simulink model "ev"  (R2021a)
settings: Solver=ode4  StartTime=0  StopTime=1082  FixedStep=sim_dt  RelTol=1e-3
model workspace (MAT data in the model file):
  T_eff_bp = [-270; -210; -150; -90; -30; 30; 90; 150; 210; 270]
  T_eff_bp_2 = [-270; -210; -150; -90; -30; 30; 90; 150; 210; 270]
  losses_table = [108927.107777 7820.2782368 7820.17609997 7820.2782368 7820.2782368 7820.2782368 7820.2782368 7820.26172359 7820.2782368 9345.38006027 108927.107777 7820.2782368 ... (100 elements, 10x10)]
  losses_table_2 = [108927.107777 7820.2782368 7820.17609997 7820.2782368 7820.2782368 7820.2782368 7820.2782368 7820.26172359 7820.2782368 9345.38006027 108927.107777 7820.2782368 ... (100 elements, 10x10)]
  w_eff_bp = [0; 888.888888889; 1777.77777778; 2666.66666667; 3555.55555556; 4444.44444444; 5333.33333333; 6222.22222222; 7111.11111111; 8000]
  w_eff_bp_2 = [0; 888.888888889; 1777.77777778; 2666.66666667; 3555.55555556; 4444.44444444; 5333.33333333; 6222.22222222; 7111.11111111; 8000]
undefined symbols (not defined in the file): Af, alpha, Bt, C, C_fa, C_free, C_sa_bat, C_sa_uc, Cd, Cmax, Continuous, Crr, DoD, effi, etaFD, etaG, FD, G, gear, Iucmax, m, M1m, M2m, Max, npar, npar_free, npara, nparf, nparfa, nparsa_bat, nparsa_UC, nser, nser_free, nserfa, nsersa_bat, nsersa_UC, Qbat, regenmax, Ri_BP, RL, ro, Rsc, Rsc_A, Rsc_F, Rsc_sa_bat, Rsc_sa_uc, rw, sim_dt, SOC_BP, SoCbatmax, SoCbatmin, SoCucmax, SoCucmin, speed, torque, VinBat, Voc_BP, Vuc, Vuc_fa, Vuc_free ... (+2)
libraries: autolibshared x41, simulink x26, autolibdcdc x13, autolibdatasheetbattery x7, autolibmappedmotor x6, fl_lib x3, nesl_utility x3, spsSupercapacitorLib x3, pid_lib x1
(part 4 of 18)

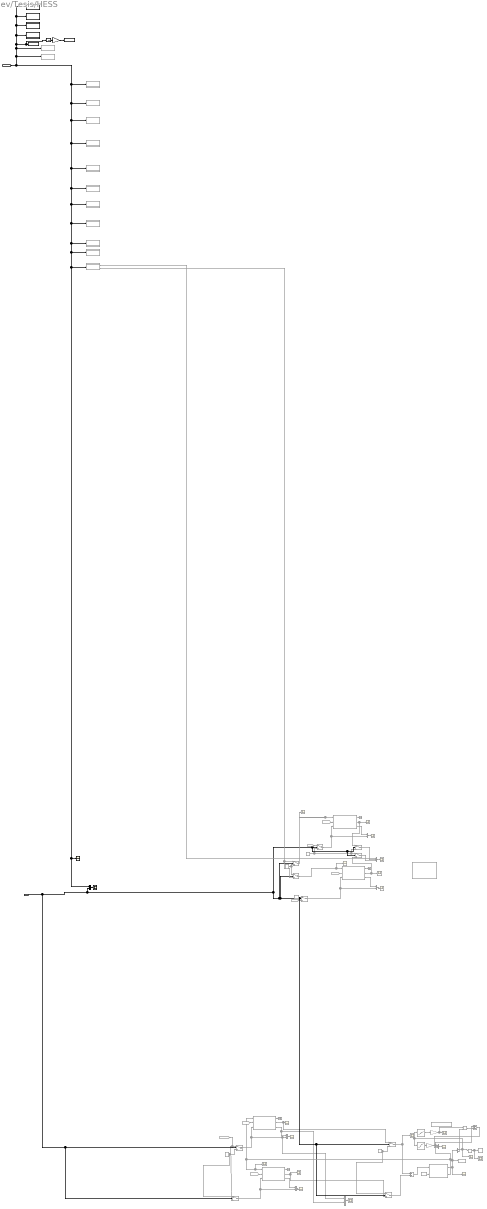
== system ev/Tesis/HESS ==
  motor power required : Inport
  motor power contr : Inport  Port=2
  Add1 : Sum  Commented=on
  Add2 : Sum  Commented=on  Inputs=+-
  Battery model : Subsystem  Commented=on
  Battery with DC/DC : Subsystem  Commented=on
  Bidirectional DC-DC : autolibdcdc/Bidirectional DC-DC  Commented=on  Tc=1/1000  Vinit=0  Plimit=100000  param_loss=Single efficiency measurement  eff=98  v_loss_bp=[0 200 400 600 800 1000]  i_loss_bp=[0 25 50 75 100]  losses_table=[100 100 100 100 100;100 150 200 250 300;100 200 300 400 500;100 250 400 550 700;100 300 500 700 900;100 350 600 850 1100]  v_eff_bp=[200 400 600 800 1000]  i_eff_bp=[25 50 75 100]  efficiency_table=[96.2 98.1 98.7 99;98.1 99 99.4 99.5;98.7 99.4 99.6 99.7;99 99.5 99.7 99.8;99.2 99.6 99.7 99.8]  x_v_bp=[-1000 -800 -600 -400 -200 200 400 600 800 1000]  x_i_bp=[-100 -75 -50 -25 25 50 75 100]  x_losses_mat=[200.400801603196 225.67703109328 200.803212851408 201.612903225806 199.999999999997 200 225 200;160.320641282556 180.541624874624 201.005025125625 202.020202020203 200 200 180 160;180.541624874624 180.722891566267 181.086519114686 197.568389057748 194.999999999999 179.999999999997 180 180;201.005025125625 181.086519114686 202.020202020203 193.67991845056 190 200 179.999999999997 200;202.020202020203 197.568389057748 193.67991845056 197.505197505197 190 190 194.999999999999 200;200 194.999999999999 190 190 197.505197505197 193.67991845056 197.568389057748 202.020202020203;200 179.999999999997 200 190 193.67991845056 202.020202020203 181.086519114686 201.005025125625;180 180 179.999999999997 194.999999999999 197.568389057748 181.086519114686 180.722891566267 180.541624874624;160 180 200 200 202.020202020203 201.005025125625 180.541624874624 160.320641282556;200 225 200 199.999999999997 201.612903225806 200.803212851408 225.67703109328 200.400801603196]  RefBlkName='autolibdcdc/Bidirectional DC-DC'
      settings: SourceProductBaseCode=PW
  Bus Selector1 : BusSelector  Commented=on  OutputSignals=BattSoc,BattCurr
  Capacitor ideal : Subsystem  Commented=on
  Capacitor real : Subsystem  Commented=on
  Capacitor semi ideal : Subsystem  Commented=on
  Capacitor semi ideal1 : Subsystem  Commented=on
  Compare To Constant2 : simulink/Logic and Bit Operations/Compare To Constant  Commented=on  relop=<=  const=0.2  OutDataTypeStr=boolean
  Constant{3..6} (4 alike) : Constant  Commented=on  Value=0
  Constant7 : Constant  Commented=on  Value=293.15
  Constant8 : Constant  Commented=on  Value=nan
  Datasheet Battery1 : autolibdatasheetbattery/Datasheet Battery  Commented=on  CapacityCtrl=Parameter  OutputVlt=Unfiltered  BattChargeMax=Qbat  Em=Voc_BP  CapLUTBp=SOC_BP  RInt=iR_bp  BattTempBp=Temp_bp  CapSOCBp=SOC_BP  Ns=nser  Np=npar  BattCapInit=Qbat*(1-DoD)  Tc=0.01  Vinit=3.3342*nser  RefBlkName='autolibdatasheetbattery/Datasheet Battery'
      settings: SourceProductBaseCode=PW
  Display2 : DisplayBlock  Commented=on  LabelPosition=Hide  Format=short  Transparency=1
  Free : Subsystem
  From{1,3..4,6} (4 alike) : From  Commented=on  GotoTag=mtr_speed  TagVisibility=global
  From2 : From  Commented=on  GotoTag=mtr_trq_corr  TagVisibility=global
  From5 : From  Commented=on  GotoTag=mtr_trq_corr  TagVisibility=global
  From8 : From  Commented=on  GotoTag=mtr_trq_corr  TagVisibility=global
  Full active1 : Subsystem  Commented=on
  Full active2 : Subsystem  Commented=on
  Full active3 : Subsystem  Commented=on
  Full active4 : Subsystem  Commented=on
  Full_active : Subsystem
  Gain6 : Gain  Commented=on  Gain=nser
  Gain7 : Gain  Commented=on  Gain=nser/npar
  Gain9 : Gain  Gain=1/(3600)
  Integrator4 : Integrator
  Mapped Motor1 : autolibmappedmotor/Mapped Motor  Commented=on  port_config=Speed  param_by=Tabulated torque-speed envelope  w_t=M1m'  T_t=M2m'  torque_max=.1  power_max=30  Tc=0.02  param_loss=Tabulated loss data  eff=100  w_eff=375  T_eff=0.08  Piron=0  Pbase=0  w_eff_bp=speed*(pi/30)  T_eff_bp=-torque  Temp_eff_bp=[233.15 293.15 373.15]  losses_table=loss_pow'  losses_table_3d=cat(3,[1.49 1.67 2.21 3.10; 0.42 0.69 1.14 2.03; 0.06 0.24 0.78 1.68; 0.42 0.69 1.14 2.03; 1.49 1.67 2.21 3.10],[1.49 1.67 2.21 3.10; 0.42 0.69 1.14 2.03; 0.06 0.24 0.78 1.68; 0.42 0.69 1.14 2.03; 1.49 1.67 2.21 3.10],[1.49 1.67 2.21 3.10; 0.42 0.69 1.14 2.03; 0.06 0.24 0.78 1.68; 0.42 0.69 1.14 2.03; 1.49 1.67 2.21 3.10])  efficiency_table=loss_pow  efficiency_table_3d=cat(3,[95 95 95 95; 95 95 95 95; 95 95 95 95; 95 95 95 95; 95 95 95 95],[95 95 95 95; 95 95 95 95; 95 95 95 95; 95 95 95 95; 95 95 95 95],[95 95 95 95; 95 95 95 95; 95 95 95 95; 95 95 95 95; 95 95 95 95])  J=2.825e-002  b=0.2564  omega_o=0  T_t_extended=[120.249620040167 121.840837540031 123.029026217228 125.013569994029 127.39293274711 130.568650599794 133.346564077512 135.328122455626 137.708231558378 139.690536286164 142.072138088259 144.453739890354 146.832356293763 150.009566845791 152.388929598871 155.168335775932 159.539705802529 161.917575856267 165.494083482603 169.069098409597 173.041917711556 176.617678988221 180.1904548662 183.766216142865 186.944173044564 188.927970471693 191.31031862346 193.692666775227 196.074268577322 197.660261629485 199.644059056614 200.831501384139 202.41152363893 203.261615914889 203.261615914889 202.41152363893 200.831501384139 199.644059056614 197.660261629485 196.074268577322 193.692666775227 191.31031862346 188.927970471693 186.944173044564 183.766216142865 180.1904548662 176.617678988221 173.041917711556 169.069098409597 165.494083482603 161.917575856267 159.539705802529 155.168335775932 152.388929598871 150.009566845791 146.832356293763 144.453739890354 142.072138088259 139.690536286164 137.708231558378 135.328122455626 133.346564077512 130.568650599794 127.39293274711 125.013569994029 123.029026217228 121.840837540031 120.249620040167]  w_t_extended=[-899.138721392584 -895.216633185855 -885.411412669033 -874.625670100529 -858.937317273614 -842.268442395016 -826.580089568101 -811.872258792868 -797.164428017635 -783.437119294084 -770.690332622215 -757.943545950346 -741.274671071749 -726.566840296516 -710.8784874696 -697.151178746049 -680.482303867452 -662.832906937172 -649.105598213621 -633.417245386706 -616.748370508109 -602.040539732875 -583.410620750913 -568.702789975681 -554.975481252129 -543.209216631943 -531.442952011757 -519.67668739157 -506.929900719701 -496.144158151197 -484.37789353101 -473.592150962506 -454.962231980544 -0.980522051682199 0.980522051682199 454.962231980544 473.592150962506 484.37789353101 496.144158151197 506.929900719701 519.67668739157 531.442952011757 543.209216631943 554.975481252129 568.702789975681 583.410620750913 602.040539732875 616.748370508109 633.417245386706 649.105598213621 662.832906937172 680.482303867452 697.151178746049 710.8784874696 726.566840296516 741.274671071749 757.943545950346 770.690332622215 783.437119294084 797.164428017635 811.872258792868 826.580089568101 842.268442395016 858.937317273614 874.625670100529 885.411412669033 895.216633185855 899.138721392584]  KLossIron=0  KLossCopper=0  x_w_eff_vec=[-837.758040957278 -816.814089933346 -795.870138909414 -774.926187885482 -753.98223686155 -733.038285837618 -712.094334813686 -691.150383789754 -670.206432765822 -649.26248174189 -628.318530717959 -607.374579694027 -586.430628670095 -565.486677646163 -544.542726622231 -523.598775598299 -502.654824574367 -481.710873550435 -460.766922526503 -439.822971502571 -418.879020478639 -397.935069454707 -376.991118430775 -356.047167406843 -335.103216382911 -314.159265358979 -293.215314335047 -272.271363311115 -251.327412287183 -230.383461263251 -209.43951023932 -188.495559215388 -167.551608191456 -146.607657167524 -125.663706143592 -104.71975511966 -83.7758040957278 -62.8318530717959 -41.8879020478639 -20.943951023932 0 20.943951023932 41.8879020478639 62.8318530717959 83.7758040957278 104.71975511966 125.663706143592 146.607657167524 167.551608191456 188.495559215388 209.43951023932 230.383461263251 251.327412287183 272.271363311115 293.215314335047 314.159265358979 335.103216382911 356.047167406843 376.991118430775 397.935069454707 418.879020478639 439.822971502571 460.766922526503 481.710873550435 502.654824574367 523.598775598299 544.542726622231 565.486677646163 586.430628670095 607.374579694027 628.318530717959 649.26248174189 670.206432765822 691.150383789754 712.094334813686 733.038285837618 753.98223686155 774.926187885482 795.870138909414 816.814089933346 837.758040957278]  x_T_eff_vec=[-270;-265;-260;-255;-250;-245;-240;-235;-230;-225;-220;-215;-210;-205;-200;-195;-190;-185;-180;-175;-170;-165;-160;-155;-150;-145;-140;-135;-130;-125;-120;-115;-110;-105;-100;-95;-90;-85;-80;-75;-70;-65;-60;-55;-50;-45;-40;-35;-30;-25;-20;-15;-12.5;-10;-5;0;5;10;12.5;15;20;25;30;35;40;45;50;55;60;65;70;75;80;85;90;95;100;105;110;115;120;125;130;135;140;145;150;155;160;165;170;175;180;185;190;195;200;205;210;215;220;225;230;235;240;245;250;255;260;265;270]  x_tmp_eff_vec=[-0.09 -0.06 -0.03 0 0.03 0.06 0.09]  x_losses_mat=[38453.09408 28860.76451 23959.87997 21362.83004 12566.37061 12315.0432 12063.71579 11812.38838 11561.06097 11309.73355 11058.40614 10807.07873 10555.75132 10304.4239 10053.09649 9801.769079 9550.441667 9299.114255 9047.786842 8796.45943 8545.132018 8293.804605 8042.477193 7791.149781 7539.822369 7288.494956 7037.167544 6785.840132 6534.512719 6283.185307 6031.857895 5780.530483 5529.20307 5277.875658 5026.548246 4775.220833 4523.893421 4272.566009 4021.238597 3769.911184 3518.583772 3267.25636 3015.928947 2764.601535 2722.713633 3015.928947 2848.377339 2932.153143 2764.601535 2722.713633 2513.274123 2513.274123 10471.97551 8377.58041 4188.790205 108121.08961086 4188.790205 8377.58041 10471.97551 2513.274123 2513.274123 2722.713633 2764.601535 2932.153143 2848.377339 3015.928947 2722.713633 2764.601535 3015.928947 3267.25636 3518.583772 3769.911184 4021.238597 4272.566009 4523.893421 4775.220833 5026.548246 5277.875658 5529.20307 5780.530483 6031.857895 6283.185307 6534.512719 6785.840132 7037.167544 7288.494956 7539.822369 7791.149781 8042.477193 8293.804605 8545.132018 8796.45943 9047.786842 9299.114255 9550.441667 9801.769079 10053.09649 10304.4239 10555.75132 10807.07873 11058.40614 11309.73355 11561.06097 11812.38838 12063.71579 12315.0432 12566.37061 21362.83004 23959.87997 28860.76451 38453.09408;37491.76673 28139.2454 23360.88297 20828.75929 12252.21135 12007.16712 11762.1229 11517.07867 11272.03444 11026.99021 10781.94599 10536.90176 9434.202739 9209.578864 8984.954989 8760.331115 8535.70724 8311.083365 8086.45949 7861.835616 7637.211741 7412.587866 7187.963991 6963.340117 6738.716242 5921.902152 5717.69863 5513.495107 5309.291585 6126.105675 5881.061448 5636.017221 5390.972994 5145.928767 4900.88454 4655.840313 4410.796086 4165.751859 3920.707632 3675.663405 3430.619178 3185.574951 2940.530724 2695.486497 2654.645792 2940.530724 2613.805088 2858.849315 2572.964383 2654.645792 2450.44227 2450.44227 10210.17612 8168.140899 4084.07045 108121.08961086 4084.07045 8168.140899 10210.17612 2450.44227 2450.44227 2654.645792 2572.964383 2858.849315 2613.805088 2940.530724 2654.645792 2695.486497 2940.530724 3185.574951 3430.619178 3675.663405 3920.707632 4165.751859 4410.796086 4655.840313 4900.88454 5145.928767 5390.972994 5636.017221 5881.061448 6126.105675 5309.291585 5513.495107 5717.69863 5921.902152 6738.716242 6963.340117 7187.963991 7412.587866 7637.211741 7861.835616 8086.45949 8311.083365 8535.70724 8760.331115 8984.954989 9209.578864 9434.202739 10536.90176 10781.94599 11026.99021 11272.03444 11517.07867 11762.1229 12007.16712 12252.21135 20828.75929 23360.88297 28139.2454 37491.76673;36530.43938 27417.72629 22761.88597 20294.68854 11938.05208 11699.29104 11460.53 11221.76896 10983.00792 10744.24688 10505.48583 9411.164393 9192.300104 8973.435816 8754.571528 8535.70724 8316.842952 8097.978663 7879.114375 7660.250087 7441.385799 7222.521511 7003.657222 6784.792934 5969.026042 5770.058507 5571.090972 5372.123438 5173.155903 4974.188368 5730.265 5491.503958 5252.742917 5013.981875 4775.220833 4536.459792 4297.69875 4058.937708 3820.176667 3581.415625 3342.654583 3103.893542 2865.1325 2626.371458 2586.577951 2865.1325 2546.784445 2785.545486 2506.990938 2586.577951 2387.610417 2387.610417 9948.376736 7958.701389 3979.350695 108121.08961086 3979.350695 7958.701389 9948.376736 2387.610417 2387.610417 2586.577951 2506.990938 2785.545486 2546.784445 2865.1325 2586.577951 2626.371458 2865.1325 3103.893542 3342.654583 3581.415625 3820.176667 4058.937708 4297.69875 4536.459792 4775.220833 5013.981875 5252.742917 5491.503958 5730.265 4974.188368 5173.155903 5372.123438 5571.090972 5770.058507 5969.026042 6784.792934 7003.657222 7222.521511 7441.385799 7660.250087 7879.114375 8097.978663 8316.842952 8535.70724 8754.571528 8973.435816 9192.300104 9411.164393 10505.48583 10744.24688 10983.00792 11221.76896 11460.53 11699.29104 11938.05208 20294.68854 22761.88597 27417.72629 36530.43938;35569.11202 26696.20717 22162.88897 ...(+103666 chars)]  x_losses_mat_3d=[37.8947368421052 25.2631578947368 12.6315789473684 0 12 24 36;18.9473684210526 12.6315789473684 6.3157894736842 0 5.99999999999999 12 18;0 0 0 0 0 0 0;18 12 5.99999999999999 0 6.3157894736842 12.6315789473684 18.9473684210526;36 24 12 0 12.6315789473684 25.2631578947368 37.8947368421052]  CalLossMapData={'BaseCageProjectFileName','';'BaseMbcProjectFileName','MbcPrj_1.mat';'TaskName','Calibrate Motor Loss Map';'ChildTasks',{{'DataName','MappedMotor-Loss_1';'TaskName','Import Loss Data'},{'TaskName','Generate Response Models'},{'TaskName','Generate Calibration'},{'TaskName','Update Block Parameters'}}}  CalLossWithTempMapData={}  aMode=1  RefBlkName='autolibmappedmotor/Mapped Motor'
      settings: SourceProductBaseCode=PW,DR,MT,UV,VE
  Mapped Motor2 : autolibmappedmotor/Mapped Motor  Commented=on  port_config=Speed  param_by=Tabulated torque-speed envelope  w_t=M1m'  T_t=M2m'  torque_max=.1  power_max=30  Tc=0.02  param_loss=Tabulated loss data  eff=100  w_eff=375  T_eff=0.08  Piron=0  Pbase=0  w_eff_bp=speed*(pi/30)  T_eff_bp=-torque  Temp_eff_bp=[233.15 293.15 373.15]  losses_table=loss_pow'  losses_table_3d=cat(3,[1.49 1.67 2.21 3.10; 0.42 0.69 1.14 2.03; 0.06 0.24 0.78 1.68; 0.42 0.69 1.14 2.03; 1.49 1.67 2.21 3.10],[1.49 1.67 2.21 3.10; 0.42 0.69 1.14 2.03; 0.06 0.24 0.78 1.68; 0.42 0.69 1.14 2.03; 1.49 1.67 2.21 3.10],[1.49 1.67 2.21 3.10; 0.42 0.69 1.14 2.03; 0.06 0.24 0.78 1.68; 0.42 0.69 1.14 2.03; 1.49 1.67 2.21 3.10])  efficiency_table=loss_pow  efficiency_table_3d=cat(3,[95 95 95 95; 95 95 95 95; 95 95 95 95; 95 95 95 95; 95 95 95 95],[95 95 95 95; 95 95 95 95; 95 95 95 95; 95 95 95 95; 95 95 95 95],[95 95 95 95; 95 95 95 95; 95 95 95 95; 95 95 95 95; 95 95 95 95])  J=2.825e-002  b=0.2564  omega_o=0  T_t_extended=[120.249620040167 121.840837540031 123.029026217228 125.013569994029 127.39293274711 130.568650599794 133.346564077512 135.328122455626 137.708231558378 139.690536286164 142.072138088259 144.453739890354 146.832356293763 150.009566845791 152.388929598871 155.168335775932 159.539705802529 161.917575856267 165.494083482603 169.069098409597 173.041917711556 176.617678988221 180.1904548662 183.766216142865 186.944173044564 188.927970471693 191.31031862346 193.692666775227 196.074268577322 197.660261629485 199.644059056614 200.831501384139 202.41152363893 203.261615914889 203.261615914889 202.41152363893 200.831501384139 199.644059056614 197.660261629485 196.074268577322 193.692666775227 191.31031862346 188.927970471693 186.944173044564 183.766216142865 180.1904548662 176.617678988221 173.041917711556 169.069098409597 165.494083482603 161.917575856267 159.539705802529 155.168335775932 152.388929598871 150.009566845791 146.832356293763 144.453739890354 142.072138088259 139.690536286164 137.708231558378 135.328122455626 133.346564077512 130.568650599794 127.39293274711 125.013569994029 123.029026217228 121.840837540031 120.249620040167]  w_t_extended=[-899.138721392584 -895.216633185855 -885.411412669033 -874.625670100529 -858.937317273614 -842.268442395016 -826.580089568101 -811.872258792868 -797.164428017635 -783.437119294084 -770.690332622215 -757.943545950346 -741.274671071749 -726.566840296516 -710.8784874696 -697.151178746049 -680.482303867452 -662.832906937172 -649.105598213621 -633.417245386706 -616.748370508109 -602.040539732875 -583.410620750913 -568.702789975681 -554.975481252129 -543.209216631943 -531.442952011757 -519.67668739157 -506.929900719701 -496.144158151197 -484.37789353101 -473.592150962506 -454.962231980544 -0.980522051682199 0.980522051682199 454.962231980544 473.592150962506 484.37789353101 496.144158151197 506.929900719701 519.67668739157 531.442952011757 543.209216631943 554.975481252129 568.702789975681 583.410620750913 602.040539732875 616.748370508109 633.417245386706 649.105598213621 662.832906937172 680.482303867452 697.151178746049 710.8784874696 726.566840296516 741.274671071749 757.943545950346 770.690332622215 783.437119294084 797.164428017635 811.872258792868 826.580089568101 842.268442395016 858.937317273614 874.625670100529 885.411412669033 895.216633185855 899.138721392584]  KLossIron=0  KLossCopper=0  x_w_eff_vec=[-837.758040957278 -816.814089933346 -795.870138909414 -774.926187885482 -753.98223686155 -733.038285837618 -712.094334813686 -691.150383789754 -670.206432765822 -649.26248174189 -628.318530717959 -607.374579694027 -586.430628670095 -565.486677646163 -544.542726622231 -523.598775598299 -502.654824574367 -481.710873550435 -460.766922526503 -439.822971502571 -418.879020478639 -397.935069454707 -376.991118430775 -356.047167406843 -335.103216382911 -314.159265358979 -293.215314335047 -272.271363311115 -251.327412287183 -230.383461263251 -209.43951023932 -188.495559215388 -167.551608191456 -146.607657167524 -125.663706143592 -104.71975511966 -83.7758040957278 -62.8318530717959 -41.8879020478639 -20.943951023932 0 20.943951023932 41.8879020478639 62.8318530717959 83.7758040957278 104.71975511966 125.663706143592 146.607657167524 167.551608191456 188.495559215388 209.43951023932 230.383461263251 251.327412287183 272.271363311115 293.215314335047 314.159265358979 335.103216382911 356.047167406843 376.991118430775 397.935069454707 418.879020478639 439.822971502571 460.766922526503 481.710873550435 502.654824574367 523.598775598299 544.542726622231 565.486677646163 586.430628670095 607.374579694027 628.318530717959 649.26248174189 670.206432765822 691.150383789754 712.094334813686 733.038285837618 753.98223686155 774.926187885482 795.870138909414 816.814089933346 837.758040957278]  x_T_eff_vec=[-270;-265;-260;-255;-250;-245;-240;-235;-230;-225;-220;-215;-210;-205;-200;-195;-190;-185;-180;-175;-170;-165;-160;-155;-150;-145;-140;-135;-130;-125;-120;-115;-110;-105;-100;-95;-90;-85;-80;-75;-70;-65;-60;-55;-50;-45;-40;-35;-30;-25;-20;-15;-12.5;-10;-5;0;5;10;12.5;15;20;25;30;35;40;45;50;55;60;65;70;75;80;85;90;95;100;105;110;115;120;125;130;135;140;145;150;155;160;165;170;175;180;185;190;195;200;205;210;215;220;225;230;235;240;245;250;255;260;265;270]  x_tmp_eff_vec=[-0.09 -0.06 -0.03 0 0.03 0.06 0.09]  x_losses_mat=[38453.09408 28860.76451 23959.87997 21362.83004 12566.37061 12315.0432 12063.71579 11812.38838 11561.06097 11309.73355 11058.40614 10807.07873 10555.75132 10304.4239 10053.09649 9801.769079 9550.441667 9299.114255 9047.786842 8796.45943 8545.132018 8293.804605 8042.477193 7791.149781 7539.822369 7288.494956 7037.167544 6785.840132 6534.512719 6283.185307 6031.857895 5780.530483 5529.20307 5277.875658 5026.548246 4775.220833 4523.893421 4272.566009 4021.238597 3769.911184 3518.583772 3267.25636 3015.928947 2764.601535 2722.713633 3015.928947 2848.377339 2932.153143 2764.601535 2722.713633 2513.274123 2513.274123 10471.97551 8377.58041 4188.790205 108121.08961086 4188.790205 8377.58041 10471.97551 2513.274123 2513.274123 2722.713633 2764.601535 2932.153143 2848.377339 3015.928947 2722.713633 2764.601535 3015.928947 3267.25636 3518.583772 3769.911184 4021.238597 4272.566009 4523.893421 4775.220833 5026.548246 5277.875658 5529.20307 5780.530483 6031.857895 6283.185307 6534.512719 6785.840132 7037.167544 7288.494956 7539.822369 7791.149781 8042.477193 8293.804605 8545.132018 8796.45943 9047.786842 9299.114255 9550.441667 9801.769079 10053.09649 10304.4239 10555.75132 10807.07873 11058.40614 11309.73355 11561.06097 11812.38838 12063.71579 12315.0432 12566.37061 21362.83004 23959.87997 28860.76451 38453.09408;37491.76673 28139.2454 23360.88297 20828.75929 12252.21135 12007.16712 11762.1229 11517.07867 11272.03444 11026.99021 10781.94599 10536.90176 9434.202739 9209.578864 8984.954989 8760.331115 8535.70724 8311.083365 8086.45949 7861.835616 7637.211741 7412.587866 7187.963991 6963.340117 6738.716242 5921.902152 5717.69863 5513.495107 5309.291585 6126.105675 5881.061448 5636.017221 5390.972994 5145.928767 4900.88454 4655.840313 4410.796086 4165.751859 3920.707632 3675.663405 3430.619178 3185.574951 2940.530724 2695.486497 2654.645792 2940.530724 2613.805088 2858.849315 2572.964383 2654.645792 2450.44227 2450.44227 10210.17612 8168.140899 4084.07045 108121.08961086 4084.07045 8168.140899 10210.17612 2450.44227 2450.44227 2654.645792 2572.964383 2858.849315 2613.805088 2940.530724 2654.645792 2695.486497 2940.530724 3185.574951 3430.619178 3675.663405 3920.707632 4165.751859 4410.796086 4655.840313 4900.88454 5145.928767 5390.972994 5636.017221 5881.061448 6126.105675 5309.291585 5513.495107 5717.69863 5921.902152 6738.716242 6963.340117 7187.963991 7412.587866 7637.211741 7861.835616 8086.45949 8311.083365 8535.70724 8760.331115 8984.954989 9209.578864 9434.202739 10536.90176 10781.94599 11026.99021 11272.03444 11517.07867 11762.1229 12007.16712 12252.21135 20828.75929 23360.88297 28139.2454 37491.76673;36530.43938 27417.72629 22761.88597 20294.68854 11938.05208 11699.29104 11460.53 11221.76896 10983.00792 10744.24688 10505.48583 9411.164393 9192.300104 8973.435816 8754.571528 8535.70724 8316.842952 8097.978663 7879.114375 7660.250087 7441.385799 7222.521511 7003.657222 6784.792934 5969.026042 5770.058507 5571.090972 5372.123438 5173.155903 4974.188368 5730.265 5491.503958 5252.742917 5013.981875 4775.220833 4536.459792 4297.69875 4058.937708 3820.176667 3581.415625 3342.654583 3103.893542 2865.1325 2626.371458 2586.577951 2865.1325 2546.784445 2785.545486 2506.990938 2586.577951 2387.610417 2387.610417 9948.376736 7958.701389 3979.350695 108121.08961086 3979.350695 7958.701389 9948.376736 2387.610417 2387.610417 2586.577951 2506.990938 2785.545486 2546.784445 2865.1325 2586.577951 2626.371458 2865.1325 3103.893542 3342.654583 3581.415625 3820.176667 4058.937708 4297.69875 4536.459792 4775.220833 5013.981875 5252.742917 5491.503958 5730.265 4974.188368 5173.155903 5372.123438 5571.090972 5770.058507 5969.026042 6784.792934 7003.657222 7222.521511 7441.385799 7660.250087 7879.114375 8097.978663 8316.842952 8535.70724 8754.571528 8973.435816 9192.300104 9411.164393 10505.48583 10744.24688 10983.00792 11221.76896 11460.53 11699.29104 11938.05208 20294.68854 22761.88597 27417.72629 36530.43938;35569.11202 26696.20717 22162.88897 ...(+103666 chars)]  x_losses_mat_3d=[37.8947368421052 25.2631578947368 12.6315789473684 0 12 24 36;18.9473684210526 12.6315789473684 6.3157894736842 0 5.99999999999999 12 18;0 0 0 0 0 0 0;18 12 5.99999999999999 0 6.3157894736842 12.6315789473684 18.9473684210526;36 24 12 0 12.6315789473684 25.2631578947368 37.8947368421052]  CalLossMapData={'BaseCageProjectFileName','';'BaseMbcProjectFileName','MbcPrj_1.mat';'TaskName','Calibrate Motor Loss Map';'ChildTasks',{{'DataName','MappedMotor-Loss_1';'TaskName','Import Loss Data'},{'TaskName','Generate Response Models'},{'TaskName','Generate Calibration'},{'TaskName','Update Block Parameters'}}}  CalLossWithTempMapData={}  aMode=1  RefBlkName='autolibmappedmotor/Mapped Motor'
      settings: SourceProductBaseCode=PW,DR,MT,UV,VE
  Mapped Motor3 : autolibmappedmotor/Mapped Motor  Commented=on  port_config=Speed  param_by=Tabulated torque-speed envelope  w_t=M1m'  T_t=-M2m'  torque_max=.1  power_max=30  Tc=0.02  param_loss=Tabulated loss data  eff=100  w_eff=375  T_eff=0.08  Piron=0  Pbase=0  w_eff_bp=w_eff_bp  T_eff_bp=T_eff_bp  Temp_eff_bp=[233.15 293.15 373.15]  losses_table=losses_table  losses_table_3d=cat(3,[1.49 1.67 2.21 3.10; 0.42 0.69 1.14 2.03; 0.06 0.24 0.78 1.68; 0.42 0.69 1.14 2.03; 1.49 1.67 2.21 3.10],[1.49 1.67 2.21 3.10; 0.42 0.69 1.14 2.03; 0.06 0.24 0.78 1.68; 0.42 0.69 1.14 2.03; 1.49 1.67 2.21 3.10],[1.49 1.67 2.21 3.10; 0.42 0.69 1.14 2.03; 0.06 0.24 0.78 1.68; 0.42 0.69 1.14 2.03; 1.49 1.67 2.21 3.10])  efficiency_table=loss_pow  efficiency_table_3d=cat(3,[95 95 95 95; 95 95 95 95; 95 95 95 95; 95 95 95 95; 95 95 95 95],[95 95 95 95; 95 95 95 95; 95 95 95 95; 95 95 95 95; 95 95 95 95],[95 95 95 95; 95 95 95 95; 95 95 95 95; 95 95 95 95; 95 95 95 95])  J=2.825e-002  b=0.2564  omega_o=0  T_t_extended=[-120.249620040167 -121.840837540031 -123.029026217228 -125.013569994029 -127.39293274711 -130.568650599794 -133.346564077512 -135.328122455626 -137.708231558378 -139.690536286164 -142.072138088259 -144.453739890354 -146.832356293763 -150.009566845791 -152.388929598871 -155.168335775932 -159.539705802529 -161.917575856267 -165.494083482603 -169.069098409597 -173.041917711556 -176.617678988221 -180.1904548662 -183.766216142865 -186.944173044564 -188.927970471693 -191.31031862346 -193.692666775227 -196.074268577322 -197.660261629485 -199.644059056614 -200.831501384139 -202.41152363893 -203.261615914889 -203.261615914889 -202.41152363893 -200.831501384139 -199.644059056614 -197.660261629485 -196.074268577322 -193.692666775227 -191.31031862346 -188.927970471693 -186.944173044564 -183.766216142865 -180.1904548662 -176.617678988221 -173.041917711556 -169.069098409597 -165.494083482603 -161.917575856267 -159.539705802529 -155.168335775932 -152.388929598871 -150.009566845791 -146.832356293763 -144.453739890354 -142.072138088259 -139.690536286164 -137.708231558378 -135.328122455626 -133.346564077512 -130.568650599794 -127.39293274711 -125.013569994029 -123.029026217228 -121.840837540031 -120.249620040167]  w_t_extended=[-899.138721392584 -895.216633185855 -885.411412669033 -874.625670100529 -858.937317273614 -842.268442395016 -826.580089568101 -811.872258792868 -797.164428017635 -783.437119294084 -770.690332622215 -757.943545950346 -741.274671071749 -726.566840296516 -710.8784874696 -697.151178746049 -680.482303867452 -662.832906937172 -649.105598213621 -633.417245386706 -616.748370508109 -602.040539732875 -583.410620750913 -568.702789975681 -554.975481252129 -543.209216631943 -531.442952011757 -519.67668739157 -506.929900719701 -496.144158151197 -484.37789353101 -473.592150962506 -454.962231980544 -0.980522051682199 0.980522051682199 454.962231980544 473.592150962506 484.37789353101 496.144158151197 506.929900719701 519.67668739157 531.442952011757 543.209216631943 554.975481252129 568.702789975681 583.410620750913 602.040539732875 616.748370508109 633.417245386706 649.105598213621 662.832906937172 680.482303867452 697.151178746049 710.8784874696 726.566840296516 741.274671071749 757.943545950346 770.690332622215 783.437119294084 797.164428017635 811.872258792868 826.580089568101 842.268442395016 858.937317273614 874.625670100529 885.411412669033 895.216633185855 899.138721392584]  KLossIron=0  KLossCopper=0  x_w_eff_vec=[-8000 -7111.11111111111 -6222.22222222222 -5333.33333333333 -4444.44444444444 -3555.55555555556 -2666.66666666667 -1777.77777777778 -888.888888888889 0 888.888888888889 1777.77777777778 2666.66666666667 3555.55555555556 4444.44444444444 5333.33333333333 6222.22222222222 7111.11111111111 8000]  x_T_eff_vec=[-270;-210;-150;-90;-30;30;90;150;210;270]  x_tmp_eff_vec=[-0.09 -0.06 -0.03 0 0.03 0.06 0.09]  x_losses_mat=[9345.3800602724 9345.3800602725 9345.3800602725 9345.38006027247 9345.38006027243 9345.38006027236 9345.38006027226 9345.38006027247 9345.38006027236 9345.3800602725;7820.27823680138 7820.27823680138 7820.27823680138 7820.27823680138 7820.27823680138 7820.27823680138 7820.27823680138 7820.27823680138 7820.27823680138 7820.27823680138;7820.26172358984 7820.26172358984 7820.26172358984 7820.26172358984 7820.26172358984 7820.26172358984 7820.26172358984 7820.26172358984 7820.26172358984 7820.26172358984;7820.27823680138 7820.27823680138 7820.27823680138 7820.27823680138 7820.27823680138 7820.27823680138 7820.27823680138 7820.27823680138 7820.27823680138 7820.27823680138;7820.27823680138 7820.27823680138 7820.27823680138 7820.27823680138 7820.27823680138 7820.27823680138 7820.27823680138 7820.27823680138 7820.27823680138 7820.27823680138;7820.27823680138 7820.27823680138 7820.27823680138 7820.27823680138 7820.27823680138 7820.27823680138 7820.27823680138 7820.27823680138 7820.27823680138 7820.27823680138;7820.27823680138 7820.27823680138 7820.27823680138 7820.27823680138 7820.27823680138 7820.27823680138 7820.27823680138 7820.27823680138 7820.27823680138 7820.27823680138;7820.17609997384 7820.17609997384 7820.17609997384 7820.17609997384 7820.17609997384 7820.17609997384 7820.17609997384 7820.17609997384 7820.17609997384 7820.17609997384;7820.27823680138 7820.27823680138 7820.27823680138 7820.27823680138 7820.27823680138 7820.27823680138 7820.27823680138 7820.27823680138 7820.27823680138 7820.27823680138;108927.107776947 108927.107776947 108927.107776947 108927.107776947 108927.107776947 108927.107776947 108927.107776947 108927.107776947 108927.107776947 108927.107776946;7820.27823680138 7820.27823680138 7820.27823680138 7820.27823680138 7820.27823680138 7820.27823680138 7820.27823680138 7820.27823680138 7820.27823680138 7820.27823680138;7820.17609997384 7820.17609997384 7820.17609997384 7820.17609997384 7820.17609997384 7820.17609997384 7820.17609997384 7820.17609997384 7820.17609997384 7820.17609997384;7820.27823680138 7820.27823680138 7820.27823680138 7820.27823680138 7820.27823680138 7820.27823680138 7820.27823680138 7820.27823680138 7820.27823680138 7820.27823680138;7820.27823680138 7820.27823680138 7820.27823680138 7820.27823680138 7820.27823680138 7820.27823680138 7820.27823680138 7820.27823680138 7820.27823680138 7820.27823680138;7820.27823680138 7820.27823680138 7820.27823680138 7820.27823680138 7820.27823680138 7820.27823680138 7820.27823680138 7820.27823680138 7820.27823680138 7820.27823680138;7820.27823680138 7820.27823680138 7820.27823680138 7820.27823680138 7820.27823680138 7820.27823680138 7820.27823680138 7820.27823680138 7820.27823680138 7820.27823680138;7820.26172358984 7820.26172358984 7820.26172358984 7820.26172358984 7820.26172358984 7820.26172358984 7820.26172358984 7820.26172358984 7820.26172358984 7820.26172358984;7820.27823680138 7820.27823680138 7820.27823680138 7820.27823680138 7820.27823680138 7820.27823680138 7820.27823680138 7820.27823680138 7820.27823680138 7820.27823680138;9345.3800602725 9345.38006027236 9345.38006027247 9345.38006027226 9345.38006027236 9345.38006027243 9345.38006027247 9345.3800602725 9345.3800602725 9345.3800602724]  x_losses_mat_3d=[37.8947368421052 25.2631578947368 12.6315789473684 0 12 24 36;18.9473684210526 12.6315789473684 6.3157894736842 0 5.99999999999999 12 18;0 0 0 0 0 0 0;18 12 5.99999999999999 0 6.3157894736842 12.6315789473684 18.9473684210526;36 24 12 0 12.6315789473684 25.2631578947368 37.8947368421052]  CalLossMapData={'BaseCageProjectFileName','CagePrj_1.cag';'BaseMbcProjectFileName','MbcPrj_1.mat';'TaskName','Calibrate Motor Loss Map';'ChildTasks',{{'DataName','MappedMotor-Loss : MappedMotor-Loss';'TaskName','Import Loss Data'},{'TaskName','Generate Response Models'},{'TaskName','Generate Calibration'},{'TaskName','Update Block Parameters'}}}  CalLossWithTempMapData={}  aMode=1  RefBlkName='autolibmappedmotor/Mapped Motor'
      settings: SourceProductBaseCode=PW,DR,MT,UV,VE
  Mapped Motor4 : autolibmappedmotor/Mapped Motor  Commented=on  port_config=Speed  param_by=Tabulated torque-speed envelope  w_t=M1m'  T_t=-M2m'  torque_max=.1  power_max=30  Tc=0.02  param_loss=Tabulated loss data  eff=100  w_eff=375  T_eff=0.08  Piron=0  Pbase=0  w_eff_bp=speed*(pi/30)  T_eff_bp=-torque  Temp_eff_bp=[233.15 293.15 373.15]  losses_table=loss_pow'  losses_table_3d=cat(3,[1.49 1.67 2.21 3.10; 0.42 0.69 1.14 2.03; 0.06 0.24 0.78 1.68; 0.42 0.69 1.14 2.03; 1.49 1.67 2.21 3.10],[1.49 1.67 2.21 3.10; 0.42 0.69 1.14 2.03; 0.06 0.24 0.78 1.68; 0.42 0.69 1.14 2.03; 1.49 1.67 2.21 3.10],[1.49 1.67 2.21 3.10; 0.42 0.69 1.14 2.03; 0.06 0.24 0.78 1.68; 0.42 0.69 1.14 2.03; 1.49 1.67 2.21 3.10])  efficiency_table=loss_pow  efficiency_table_3d=cat(3,[95 95 95 95; 95 95 95 95; 95 95 95 95; 95 95 95 95; 95 95 95 95],[95 95 95 95; 95 95 95 95; 95 95 95 95; 95 95 95 95; 95 95 95 95],[95 95 95 95; 95 95 95 95; 95 95 95 95; 95 95 95 95; 95 95 95 95])  J=2.825e-002  b=0.2564  omega_o=0  T_t_extended=[-120.249620040167 -121.840837540031 -123.029026217228 -125.013569994029 -127.39293274711 -130.568650599794 -133.346564077512 -135.328122455626 -137.708231558378 -139.690536286164 -142.072138088259 -144.453739890354 -146.832356293763 -150.009566845791 -152.388929598871 -155.168335775932 -159.539705802529 -161.917575856267 -165.494083482603 -169.069098409597 -173.041917711556 -176.617678988221 -180.1904548662 -183.766216142865 -186.944173044564 -188.927970471693 -191.31031862346 -193.692666775227 -196.074268577322 -197.660261629485 -199.644059056614 -200.831501384139 -202.41152363893 -203.261615914889 -203.261615914889 -202.41152363893 -200.831501384139 -199.644059056614 -197.660261629485 -196.074268577322 -193.692666775227 -191.31031862346 -188.927970471693 -186.944173044564 -183.766216142865 -180.1904548662 -176.617678988221 -173.041917711556 -169.069098409597 -165.494083482603 -161.917575856267 -159.539705802529 -155.168335775932 -152.388929598871 -150.009566845791 -146.832356293763 -144.453739890354 -142.072138088259 -139.690536286164 -137.708231558378 -135.328122455626 -133.346564077512 -130.568650599794 -127.39293274711 -125.013569994029 -123.029026217228 -121.840837540031 -120.249620040167]  w_t_extended=[-899.138721392584 -895.216633185855 -885.411412669033 -874.625670100529 -858.937317273614 -842.268442395016 -826.580089568101 -811.872258792868 -797.164428017635 -783.437119294084 -770.690332622215 -757.943545950346 -741.274671071749 -726.566840296516 -710.8784874696 -697.151178746049 -680.482303867452 -662.832906937172 -649.105598213621 -633.417245386706 -616.748370508109 -602.040539732875 -583.410620750913 -568.702789975681 -554.975481252129 -543.209216631943 -531.442952011757 -519.67668739157 -506.929900719701 -496.144158151197 -484.37789353101 -473.592150962506 -454.962231980544 -0.980522051682199 0.980522051682199 454.962231980544 473.592150962506 484.37789353101 496.144158151197 506.929900719701 519.67668739157 531.442952011757 543.209216631943 554.975481252129 568.702789975681 583.410620750913 602.040539732875 616.748370508109 633.417245386706 649.105598213621 662.832906937172 680.482303867452 697.151178746049 710.8784874696 726.566840296516 741.274671071749 757.943545950346 770.690332622215 783.437119294084 797.164428017635 811.872258792868 826.580089568101 842.268442395016 858.937317273614 874.625670100529 885.411412669033 895.216633185855 899.138721392584]  KLossIron=0  KLossCopper=0  x_w_eff_vec=[-837.758040957278 -816.814089933346 -795.870138909414 -774.926187885482 -753.98223686155 -733.038285837618 -712.094334813686 -691.150383789754 -670.206432765822 -649.26248174189 -628.318530717959 -607.374579694027 -586.430628670095 -565.486677646163 -544.542726622231 -523.598775598299 -502.654824574367 -481.710873550435 -460.766922526503 -439.822971502571 -418.879020478639 -397.935069454707 -376.991118430775 -356.047167406843 -335.103216382911 -314.159265358979 -293.215314335047 -272.271363311115 -251.327412287183 -230.383461263251 -209.43951023932 -188.495559215388 -167.551608191456 -146.607657167524 -125.663706143592 -104.71975511966 -83.7758040957278 -62.8318530717959 -41.8879020478639 -20.943951023932 0 20.943951023932 41.8879020478639 62.8318530717959 83.7758040957278 104.71975511966 125.663706143592 146.607657167524 167.551608191456 188.495559215388 209.43951023932 230.383461263251 251.327412287183 272.271363311115 293.215314335047 314.159265358979 335.103216382911 356.047167406843 376.991118430775 397.935069454707 418.879020478639 439.822971502571 460.766922526503 481.710873550435 502.654824574367 523.598775598299 544.542726622231 565.486677646163 586.430628670095 607.374579694027 628.318530717959 649.26248174189 670.206432765822 691.150383789754 712.094334813686 733.038285837618 753.98223686155 774.926187885482 795.870138909414 816.814089933346 837.758040957278]  x_T_eff_vec=[-270;-265;-260;-255;-250;-245;-240;-235;-230;-225;-220;-215;-210;-205;-200;-195;-190;-185;-180;-175;-170;-165;-160;-155;-150;-145;-140;-135;-130;-125;-120;-115;-110;-105;-100;-95;-90;-85;-80;-75;-70;-65;-60;-55;-50;-45;-40;-35;-30;-25;-20;-15;-12.5;-10;-5;0;5;10;12.5;15;20;25;30;35;40;45;50;55;60;65;70;75;80;85;90;95;100;105;110;115;120;125;130;135;140;145;150;155;160;165;170;175;180;185;190;195;200;205;210;215;220;225;230;235;240;245;250;255;260;265;270]  x_tmp_eff_vec=[-0.09 -0.06 -0.03 0 0.03 0.06 0.09]  x_losses_mat=[38453.09408 28860.76451 23959.87997 21362.83004 12566.37061 12315.0432 12063.71579 11812.38838 11561.06097 11309.73355 11058.40614 10807.07873 10555.75132 10304.4239 10053.09649 9801.769079 9550.441667 9299.114255 9047.786842 8796.45943 8545.132018 8293.804605 8042.477193 7791.149781 7539.822369 7288.494956 7037.167544 6785.840132 6534.512719 6283.185307 6031.857895 5780.530483 5529.20307 5277.875658 5026.548246 4775.220833 4523.893421 4272.566009 4021.238597 3769.911184 3518.583772 3267.25636 3015.928947 2764.601535 2722.713633 3015.928947 2848.377339 2932.153143 2764.601535 2722.713633 2513.274123 2513.274123 10471.97551 8377.58041 4188.790205 108121.08961086 4188.790205 8377.58041 10471.97551 2513.274123 2513.274123 2722.713633 2764.601535 2932.153143 2848.377339 3015.928947 2722.713633 2764.601535 3015.928947 3267.25636 3518.583772 3769.911184 4021.238597 4272.566009 4523.893421 4775.220833 5026.548246 5277.875658 5529.20307 5780.530483 6031.857895 6283.185307 6534.512719 6785.840132 7037.167544 7288.494956 7539.822369 7791.149781 8042.477193 8293.804605 8545.132018 8796.45943 9047.786842 9299.114255 9550.441667 9801.769079 10053.09649 10304.4239 10555.75132 10807.07873 11058.40614 11309.73355 11561.06097 11812.38838 12063.71579 12315.0432 12566.37061 21362.83004 23959.87997 28860.76451 38453.09408;37491.76673 28139.2454 23360.88297 20828.75929 12252.21135 12007.16712 11762.1229 11517.07867 11272.03444 11026.99021 10781.94599 10536.90176 9434.202739 9209.578864 8984.954989 8760.331115 8535.70724 8311.083365 8086.45949 7861.835616 7637.211741 7412.587866 7187.963991 6963.340117 6738.716242 5921.902152 5717.69863 5513.495107 5309.291585 6126.105675 5881.061448 5636.017221 5390.972994 5145.928767 4900.88454 4655.840313 4410.796086 4165.751859 3920.707632 3675.663405 3430.619178 3185.574951 2940.530724 2695.486497 2654.645792 2940.530724 2613.805088 2858.849315 2572.964383 2654.645792 2450.44227 2450.44227 10210.17612 8168.140899 4084.07045 108121.08961086 4084.07045 8168.140899 10210.17612 2450.44227 2450.44227 2654.645792 2572.964383 2858.849315 2613.805088 2940.530724 2654.645792 2695.486497 2940.530724 3185.574951 3430.619178 3675.663405 3920.707632 4165.751859 4410.796086 4655.840313 4900.88454 5145.928767 5390.972994 5636.017221 5881.061448 6126.105675 5309.291585 5513.495107 5717.69863 5921.902152 6738.716242 6963.340117 7187.963991 7412.587866 7637.211741 7861.835616 8086.45949 8311.083365 8535.70724 8760.331115 8984.954989 9209.578864 9434.202739 10536.90176 10781.94599 11026.99021 11272.03444 11517.07867 11762.1229 12007.16712 12252.21135 20828.75929 23360.88297 28139.2454 37491.76673;36530.43938 27417.72629 22761.88597 20294.68854 11938.05208 11699.29104 11460.53 11221.76896 10983.00792 10744.24688 10505.48583 9411.164393 9192.300104 8973.435816 8754.571528 8535.70724 8316.842952 8097.978663 7879.114375 7660.250087 7441.385799 7222.521511 7003.657222 6784.792934 5969.026042 5770.058507 5571.090972 5372.123438 5173.155903 4974.188368 5730.265 5491.503958 5252.742917 5013.981875 4775.220833 4536.459792 4297.69875 4058.937708 3820.176667 3581.415625 3342.654583 3103.893542 2865.1325 2626.371458 2586.577951 2865.1325 2546.784445 2785.545486 2506.990938 2586.577951 2387.610417 2387.610417 9948.376736 7958.701389 3979.350695 108121.08961086 3979.350695 7958.701389 9948.376736 2387.610417 2387.610417 2586.577951 2506.990938 2785.545486 2546.784445 2865.1325 2586.577951 2626.371458 2865.1325 3103.893542 3342.654583 3581.415625 3820.176667 4058.937708 4297.69875 4536.459792 4775.220833 5013.981875 5252.742917 5491.503958 5730.265 4974.188368 5173.155903 5372.123438 5571.090972 5770.058507 5969.026042 6784.792934 7003.657222 7222.521511 7441.385799 7660.250087 7879.114375 8097.978663 8316.842952 8535.70724 8754.571528 8973.435816 9192.300104 9411.164393 10505.48583 10744.24688 10983.00792 11221.76896 11460.53 11699.29104 11938.05208 20294.68854 22761.88597 27417.72629 36530.43938;35569.11202 26696.20717 22162.88897 ...(+103666 chars)]  x_losses_mat_3d=[37.8947368421052 25.2631578947368 12.6315789473684 0 12 24 36;18.9473684210526 12.6315789473684 6.3157894736842 0 5.99999999999999 12 18;0 0 0 0 0 0 0;18 12 5.99999999999999 0 6.3157894736842 12.6315789473684 18.9473684210526;36 24 12 0 12.6315789473684 25.2631578947368 37.8947368421052]  CalLossMapData={'BaseCageProjectFileName','';'BaseMbcProjectFileName','MbcPrj_1.mat';'TaskName','Calibrate Motor Loss Map';'ChildTasks',{{'DataName','MappedMotor-Loss_1';'TaskName','Import Loss Data'},{'TaskName','Generate Response Models'},{'TaskName','Generate Calibration'},{'TaskName','Update Block Parameters'}}}  CalLossWithTempMapData={}  aMode=1  RefBlkName='autolibmappedmotor/Mapped Motor'
      settings: SourceProductBaseCode=PW,DR,MT,UV,VE
  Mux{1..3,5..6} (5 alike) : Mux  Commented=on  Inputs=2
  Mux11 : Mux  Inputs=2
  Mux7 : Mux  Commented=on  Inputs=3
  Mux8 : Mux  Commented=on  Inputs=3
  OCV2 : Lookup_n-D  Commented=on  NumberOfTableDimensions=1  BreakpointsForDimension1=SOC_BP  Table=Voc_BP  InternalRulePriority=Speed  RndMeth=Simplest  InputSameDT=on
  Pow : Scope
  Product2 : Product  Commented=on
  Ri2 : Lookup_n-D  Commented=on  NumberOfTableDimensions=1  BreakpointsForDimension1=SOC_BP  Table=Ri_BP  InternalRulePriority=Speed  RndMeth=Simplest  InputSameDT=on
  Scope{2..4,8..12,15..25} (19 alike) : Scope  Commented=on
  Scope38 : Scope
  Stop Simulation1 : Stop  Commented=on
  Switch{,1..4,6,8..9} (8 alike) : Switch  Commented=on
  Switch5 : Switch  Commented=on  Criteria=u2 > Threshold
  Switch7 : Switch  Commented=on  Criteria=u2 ~= 0
  Terminator{1..4} (4 alike) : Terminator  Commented=on
  To Workspace : ToWorkspace  VariableName=zz_pow  SaveFormat=Structure With Time  SampleTime=-1
  To Workspace1 : ToWorkspace  Commented=on  VariableName=Batt2  SaveFormat=Structure With Time  SampleTime=-1
  To Workspace2 : ToWorkspace  VariableName=zz_ener  SaveFormat=Structure With Time  SampleTime=-1
  battery model limited : Subsystem  Commented=on
  semi active Bat/Bat : Subsystem  Commented=on
  semi active battery/uc : Subsystem  Commented=on
  semi_active_UC : Subsystem
  semi_active_bat : Subsystem
  wires:
  Mapped Motor1/3 -> Mux2/1
  Mapped Motor1/1 -> Terminator1/1
  From3/1 -> Mapped Motor1/2
  Switch3/1 -> Mux3/2, Mapped Motor3/3
  Switch2/1 -> Mux2/2, Mapped Motor1/3
  From2/1 -> Switch2/1
  From8/1 -> Switch3/3
  Constant6/1 -> Switch3/1
  Mux2/1 -> Scope23/1
  Mapped Motor3/2 -> Switch8/3, Scope2/1
  Mapped Motor3/1 -> Terminator4/1
  Constant5/1 -> Switch7/3, Switch8/1, Switch2/3
  From1/1 -> ?
  Mux3/1 -> Scope19/1
  Mapped Motor3/3 -> Mux3/1
  Mapped Motor1/2 -> Switch7/1, Scope3/1
  From5/1 -> Switch4/3, Switch1/1
  From4/1 -> Mapped Motor4/2
  Mapped Motor4/1 -> Terminator3/1
  Switch1/1 -> Mux6/1, Mux1/2, Mapped Motor2/3
  Mapped Motor4/2 -> Switch6/3, Scope9/1
  Mux6/1 -> Scope11/1
  Mapped Motor2/1 -> Terminator2/1
  Mapped Motor2/3 -> Mux6/2, Mux1/1
  Mapped Motor4/3 -> Mux5/1
  Mux1/1 -> Scope10/1
  Constant3/1 -> Switch4/1, Switch1/3
  Switch4/1 -> Mux5/2, Mapped Motor4/3
  Mux5/1 -> Scope8/1
  From6/1 -> Mapped Motor2/2
  Mapped Motor2/2 -> Switch5/1, Scope12/1
  Constant4/1 -> Switch6/1, Switch5/3
  motor power required/1 -> Switch/2, Switch9/2, Switch5/2, Switch6/2, Switch3/2, Switch8/2, Switch7/2, Switch2/2, Mux11/2, Switch4/2, Switch1/2
  Add1/1 -> Datasheet Battery1/1
  Switch5/1 -> Scope24/1, Add1/1
  Switch6/1 -> Add1/2
  Constant7/1 -> Datasheet Battery1/2
  Add2/1 -> Mux7/3
  Ri2/1 -> Gain7/1
  Gain7/1 -> Product2/1, Scope15/1
  Gain6/1 -> Add2/1, Mux7/1
  Bus Selector1/2 -> Product2/2  "<BattCurr>"
  Mux7/1 -> Scope16/1
  Datasheet Battery1/1 -> Scope20/1, Bus Selector1/1, To Workspace1/1
  Product2/1 -> Add2/2
  OCV2/1 -> Gain6/1
  Compare To Constant2/1 -> Scope18/1, Stop Simulation1/1
  Bus Selector1/1 -> Ri2/1, OCV2/1, Scope21/1, Compare To Constant2/1  "<BattSoc>"
  Datasheet Battery1/2 -> Scope4/1, Mapped Motor4/1, Mapped Motor2/1, Mux7/2  "Voltage"
  Mux8/1 -> Scope25/1
  Switch7/1 -> Mux8/2
  Switch8/1 -> Mux8/3
  Constant8/1 -> Switch9/1, Switch/3
  Switch9/1 -> Scope17/1, Mapped Motor3/1
  Switch/1 -> Scope22/1, Mapped Motor1/1
  Mux11/1 -> Scope38/1
  Battery model/2(Voltage) -> Switch9/3, Switch/1
  Battery model/1(<BattCurr>) -> Mux8/1
  Integrator4/1 -> Gain9/1
  motor power contr/1 -> Integrator4/1, To Workspace/1, Free/1(motor_pwr_contr), semi_active_bat/1(motor_pwr_contr), semi_active_UC/1(motor_pwr_contr), Full_active/1(motor_pwr_contr), Full active4/1(motor_pwr_contr), Full active1/1(motor_pwr_contr), Full active2/1(motor_pwr_contr), Mux11/1, Pow/1, Battery model/1(motor_pwr_contr), Capacitor ideal/1(motor_pwr_contr), battery model limited/1(motor_pwr_contr), Capacitor real/1(motor_pwr_contr), Capacitor semi ideal/1(motor_pwr_contr), Capacitor semi ideal1/1(motor_pwr_contr), Battery with DC/DC/1(motor_pwr_contr), Full active3/1(motor_pwr_contr), semi active battery/uc/1(motor_pwr_contr), semi active Bat/Bat/1(motor_pwr_contr)  "Pow"
  Gain9/1 -> To Workspace2/1
